simulink model "mech_four_bar_stat"  (Simulink 7.1)
settings: Solver=ode45  StartTime=0.0  StopTime=10.0  RelTol=1e-3  AbsTol=1e-3
libraries: mblibv1 x12
settings Model: Creator=paulk  LastModifiedBy=batserve  ExtModeAutoUpdateStatusClock=off
settings DataIOCC: SignalLoggingName=sigsOut
settings OptimizationCC: BooleanDataType=off  InlineInvariantSignals=on
settings DebuggingCC: SaveWithParameterizedLinksMsg=none  CheckExecutionContextPreStartOutputMsg=on  CheckExecutionContextRuntimeOutputMsg=on  SignalResolutionControl=TryResolveAllWithWarning  SolverPrmCheckMsg=none  MultiTaskDSMMsg=warning  MultiTaskCondExecSysMsg=none  StrictBusMsg=None
settings HardwareCC: TargetBitPerLong=64  TargetEndianess=LittleEndian  TargetWordSize=64  TargetHWDeviceType=MATLAB Host  ProdEqTarget=off
settings RTWCC: SystemTargetFile=rsim.tlc  TemplateMakefile=rsim_default_tmf  Description=Rapid Simulation Target  ProcessScript=rsim_make_rtw_hook  IncludeERTFirstTime=on
settings RSimTargetCC: TargetFcnLib=ansi_tfl_tmw.mat  TargetFunctionLibrary=ANSI_C  IsPILTarget=off  EnableShiftOperators=on  PortableWordSizes=off
settings SimMechanicsCC: WarnOnRedundantConstraints=off  VisOnUpdateDiagram=on  VisDuringSimulation=on

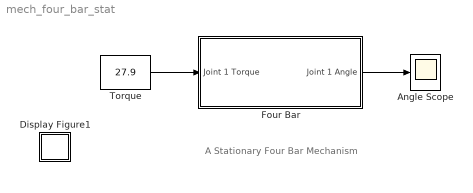
== system mech_four_bar_stat ==
  note: A Stationary Four Bar Mechanism
  Angle Scope : Scope
      settings: TimeRange=10  YMax=25
  Display Figure1 : Subsystem  Tag=Help  Description="Help callback for kinematic four bar model: mech_four_bar_kin.  Opens Help browser to Type 19 marker at documentation for this tutorial model."
      settings: OpenFcn=helpview([docroot '/toolbox/physmod/mech/mech.map'], 'mech_four_bar_stat_help');
      mask Type: Help callback
      mask Display: image(imread('info.bmp'))
  Four Bar : Subsystem
  Torque : Constant  Value=27.9  OutDataType=sfix(16)  OutScaling=2^0
  wires:
  Torque/1 -> Four Bar/1(Joint 1 Torque)
  Four Bar/1(Joint 1 Angle) -> Angle Scope/1

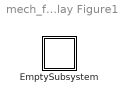
== system mech_four_bar_stat/Display Figure1 ==
  EmptySubsystem : Subsystem

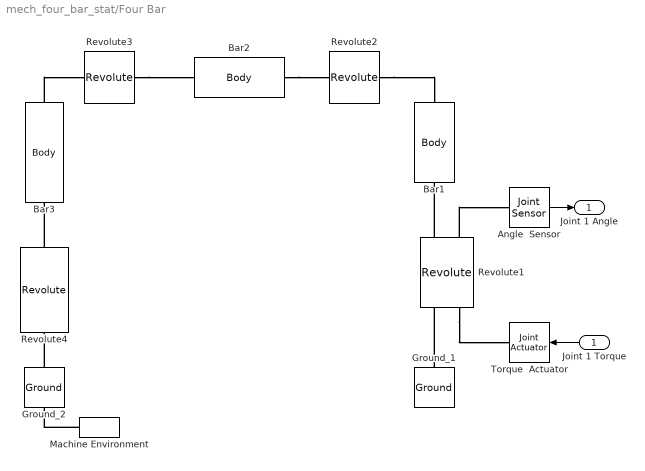
== system mech_four_bar_stat/Four Bar ==
  Joint 1 Torque : Inport  Orientation=left  OutDataType=sfix(16)  OutScaling=2^0
  Angle  Sensor : mblibv1/Sensors &  Actuators/Joint Sensor  DialogController=MECH.DynMechDlgSource  SystemSampleTime=-1  PhysicalDomain=Mechanical  PortType=blob  Muxed=on  Pose=off  Angle=on  AngleUnits=deg  ArcVelocity=off  ArcVelocityUnits=deg/s  ArcAcceleration=off  ArcAccelerationUnits=deg/s^2  CoordPosition=on  CoordPositionUnits=m  Velocity=off  VelocityUnits=m/s  Acceleration=off  AccelerationUnits=m/s^2  Quaternion=on  QuaternionDT=off  QuaternionDDT=off  QuaternionUnits=off  OutputVector=[ 1 ]  ActiveIO=on  Width=1  DialogClass=MechanicalSensorBlock  Primitive=R1  Force=off  ForceUnits=N  Torque=off  TorqueUnits=N-m  ReferenceFrame=Absolute (INERTIAL)  ReactionSensedSide=Base  ReactionReferenceFrame=Absolute (World)  ReactionForce=off  ReactionForceUnits=N  ReactionMoment=off  ReactionMomentUnits=N-m
  Bar1 : mblibv1/Bodies/Body  Orientation=up  DialogController=MECH.DynMechDlgSource  PhysicalDomain=mechanical  SubClassName=Unknown  LeftPortType=workingframe  RightPortType=workingframe  LConnTagsString=CS1  RConnTagsString=CS2  DialogClass=MechanicalBodyBlock  Mass=5.357  MassUnits=kg  InertiaUnits=kg*m^2  Inertia=[1.07e-3 0 0; 0 0.143 0;0 0 0.143]  Shape=Cylinder  ShapeDims=[1 1]  ShapeUnits=m  ShapeUse=false  Density=1  DensityUnits=kg/m^3  DensityUse=false  GraphicsMode=1  BodyColor=[0.5 0.5 0.5]  GraphicsObj=[]  AttachedToCS=1  CG=Left$CG$[0.03 0.282 0]$WORLD$CS1$m$[0 0 83.1]$Euler X-Y-Z$deg$WORLD$false  WorkingFrames=Left$CS1$[0 0 0]$WORLD$ADJOINING$m$[0 0 0]$Euler X-Y-Z$deg$WORLD$true#Right$CS2$[0.063 0.597 0]$WORLD$CS1$m$[0 0 0]$Euler X-Y-Z$deg$WORLD$true  CGPos=[0.03 0.282 0]  CGRot=[0 0 83.1]  CS0Pos=[]  CS0Rot=[]  CS1Pos=[0 0 0]  CS1Rot=[0 0 0]  CS2Pos=[0.063 0.597 0]  CS2Rot=[0 0 0]  CS3Pos=[]  CS3Rot=[]  CS4Pos=[]  CS4Rot=[]  CS5Pos=[]  CS5Rot=[]  CS6Pos=[]  CS6Rot=[]  CS7Pos=[]  CS7Rot=[]  CS8Pos=[]  CS8Rot=[]  CS9Pos=[]  CS9Rot=[]  CS10Pos=[]  CS10Rot=[]  CS11Pos=[]  CS11Rot=[]  CS12Pos=[]  CS12Rot=[]  CS13Pos=[]  CS13Rot=[]  CS14Pos=[]  CS14Rot=[]  CS15Pos=[]  CS15Rot=[]  CS16Pos=[]  CS16Rot=[]  CS17Pos=[]  CS17Rot=[]  CS18Pos=[]  CS18Rot=[]  CS19Pos=[]  CS19Rot=[]  CS20Pos=[]  CS20Rot=[]
  Bar2 : mblibv1/Bodies/Body  Orientation=left  DialogController=MECH.DynMechDlgSource  PhysicalDomain=mechanical  SubClassName=Unknown  LeftPortType=workingframe  RightPortType=workingframe  LConnTagsString=CS1  RConnTagsString=CS2  DialogClass=MechanicalBodyBlock  Mass=9.028  MassUnits=kg  InertiaUnits=kg*m^2  Inertia=[1.8e-3 0 0; 0 0.678 0;0 0 0.678]  Shape=Cylinder  ShapeDims=[1 1]  ShapeUnits=m  ShapeUse=false  Density=1  DensityUnits=kg/m^3  DensityUse=false  GraphicsMode=1  BodyColor=[0.5 0.5 0.5]  GraphicsObj=[]  AttachedToCS=1  CG=Left$CG$[-0.427 -0.242 0]$WORLD$CS1$m$[0 0 29.5]$Euler X-Y-Z$deg$WORLD$false  WorkingFrames=Left$CS1$[0 0 0]$WORLD$ADJOINING$m$[0 0 0]$Euler X-Y-Z$deg$WORLD$true#Right$CS2$[-0.87 -0.493 0]$WORLD$CS1$m$[0 0 0]$Euler X-Y-Z$deg$WORLD$true  CGPos=[-0.427 -0.242 0]  CGRot=[0 0 29.5]  CS0Pos=[]  CS0Rot=[]  CS1Pos=[0 0 0]  CS1Rot=[0 0 0]  CS2Pos=[-0.87 -0.493 0]  CS2Rot=[0 0 0]  CS3Pos=[]  CS3Rot=[]  CS4Pos=[]  CS4Rot=[]  CS5Pos=[]  CS5Rot=[]  CS6Pos=[]  CS6Rot=[]  CS7Pos=[]  CS7Rot=[]  CS8Pos=[]  CS8Rot=[]  CS9Pos=[]  CS9Rot=[]  CS10Pos=[]  CS10Rot=[]  CS11Pos=[]  CS11Rot=[]  CS12Pos=[]  CS12Rot=[]  CS13Pos=[]  CS13Rot=[]  CS14Pos=[]  CS14Rot=[]  CS15Pos=[]  CS15Rot=[]  CS16Pos=[]  CS16Rot=[]  CS17Pos=[]  CS17Rot=[]  CS18Pos=[]  CS18Rot=[]  CS19Pos=[]  CS19Rot=[]  CS20Pos=[]  CS20Rot=[]
  Bar3 : mblibv1/Bodies/Body  Orientation=down  DialogController=MECH.DynMechDlgSource  PhysicalDomain=mechanical  SubClassName=Unknown  LeftPortType=workingframe  RightPortType=workingframe  LConnTagsString=CS1  RConnTagsString=CS2  DialogClass=MechanicalBodyBlock  Mass=0.991  MassUnits=kg  InertiaUnits=kg*m^2  Inertia=[2.06e-4 0 0; 0 1.1e-3 0;0 0 1.1e-3]  Shape=Cylinder  ShapeDims=[1 1]  ShapeUnits=m  ShapeUse=false  Density=1  DensityUnits=kg/m^3  DensityUse=false  GraphicsMode=1  BodyColor=[0.5 0.5 0.5]  GraphicsObj=[]  AttachedToCS=1  CG=Left$CG$[-0.027 -0.048 0]$WORLD$CS1$m$[0 0 60]$Euler X-Y-Z$deg$WORLD$false  WorkingFrames=Left$CS1$[0 0 0]$WORLD$ADJOINING$m$[0 0 0]$Euler X-Y-Z$deg$WORLD$true#Right$CS2$[0 0 0]$WORLD$ADJOINING$m$[0 0 0]$Euler X-Y-Z$deg$WORLD$true  CGPos=[-0.027 -0.048 0]  CGRot=[0 0 60]  CS0Pos=[]  CS0Rot=[]  CS1Pos=[0 0 0]  CS1Rot=[0 0 0]  CS2Pos=[0 0 0]  CS2Rot=[0 0 0]  CS3Pos=[]  CS3Rot=[]  CS4Pos=[]  CS4Rot=[]  CS5Pos=[]  CS5Rot=[]  CS6Pos=[]  CS6Rot=[]  CS7Pos=[]  CS7Rot=[]  CS8Pos=[]  CS8Rot=[]  CS9Pos=[]  CS9Rot=[]  CS10Pos=[]  CS10Rot=[]  CS11Pos=[]  CS11Rot=[]  CS12Pos=[]  CS12Rot=[]  CS13Pos=[]  CS13Rot=[]  CS14Pos=[]  CS14Rot=[]  CS15Pos=[]  CS15Rot=[]  CS16Pos=[]  CS16Rot=[]  CS17Pos=[]  CS17Rot=[]  CS18Pos=[]  CS18Rot=[]  CS19Pos=[]  CS19Rot=[]  CS20Pos=[]  CS20Rot=[]
  Ground_1 : mblibv1/Bodies/Ground  Orientation=up  DialogController=MECH.DynMechDlgSource  SystemSampleTime=-1  LeftPortType=env  RightPortType=workingframe  PhysicalDomain=Mechanical  DialogClass=GroundBlock  CoordPosition=[0.434 0.04 0]  CoordPositionUnits=m  StateVectorMgrId=-1  MachineId=[0 0]  ShowEnvPort=off
  Ground_2 : mblibv1/Bodies/Ground  Orientation=up  DialogController=MECH.DynMechDlgSource  SystemSampleTime=-1  LeftPortType=env  RightPortType=workingframe  PhysicalDomain=Mechanical  DialogClass=GroundBlock  CoordPosition=[-0.433 0.04 0]  CoordPositionUnits=m  StateVectorMgrId=-1  MachineId=[0 0]  ShowEnvPort=on
  Machine Environment : mblibv1/Bodies/Machine Environment  Tag=Factory ground  Orientation=left  DialogController=MECH.DialogSource  SystemSampleTime=-1  PortType=env  PhysicalDomain=Mechanical  DialogTemplateClass=MECH.MachineEnvironment  SyncWhenCopied=off  Gravity=[0 -9.81 0]  GravityUnits=m/s^2  GravityAsSignal=off  Dimensionality=3D Only  AnalysisType=Forward dynamics  LinearAssemblyTolerance=1e-3  LinearAssemblyToleranceUnits=m  AngularAssemblyTolerance=1e-3  AngularAssemblyToleranceUnits=rad  ConstraintSolverType=Tolerancing  ConstraintRelTolerance=1e-4  ConstraintAbsTolerance=1e-4  UseRobustSingularityHandling=off  RedundancyAnalysisToleranceType=Automatically select tolerance  RedundancyAnalysisTolerance=1e-14  StatePerturbationType=Adaptive  PerturbationSize=0  VisualizeMachine=on
  Revolute1 : mblibv1/Joints/Revolute  Orientation=up  DialogController=MECH.DynMechDlgSource  PhysicalDomain=mechanical  SubClassName=Unknown  LeftPortType=blob  RightPortType=blob  LConnTagsString=__newl0|SA1  RConnTagsString=__newr0|SA1  NumSAPorts=2  CutJoint=off  MarkAsCut=off  Primitives=revolute  PrimitiveProps=R1$WORLD$[0 0 1]$revolute  DialogClass=JointBlock  R1Axis=[0 0 1]
  Revolute2 : mblibv1/Joints/Revolute  Orientation=left  DialogController=MECH.DynMechDlgSource  PhysicalDomain=mechanical  SubClassName=Unknown  LeftPortType=blob  RightPortType=blob  LConnTagsString=__newl0  RConnTagsString=__newr0  NumSAPorts=0  CutJoint=off  MarkAsCut=off  Primitives=revolute  PrimitiveProps=R1$WORLD$[0 0 1]$revolute  DialogClass=JointBlock  R1Axis=[0 0 1]
  Revolute3 : mblibv1/Joints/Revolute  Orientation=left  DialogController=MECH.DynMechDlgSource  PhysicalDomain=mechanical  SubClassName=Unknown  LeftPortType=blob  RightPortType=blob  LConnTagsString=__newl0  RConnTagsString=__newr0  NumSAPorts=0  CutJoint=off  MarkAsCut=off  Primitives=revolute  PrimitiveProps=R1$WORLD$[0 0 1]$revolute  DialogClass=JointBlock  R1Axis=[0 0 1]
  Revolute4 : mblibv1/Joints/Revolute  Orientation=down  DialogController=MECH.DynMechDlgSource  PhysicalDomain=mechanical  SubClassName=Unknown  LeftPortType=blob  RightPortType=blob  LConnTagsString=__newl0  RConnTagsString=__newr0  NumSAPorts=0  CutJoint=off  MarkAsCut=off  Primitives=revolute  PrimitiveProps=R1$WORLD$[0 0 1]$revolute  DialogClass=JointBlock  R1Axis=[0 0 1]
  Torque  Actuator : mblibv1/Sensors &  Actuators/Joint Actuator  Orientation=left  DialogController=MECH.DynMechDlgSource  SystemSampleTime=-1  PhysicalDomain=Mechanical  PortType=blob  ActuationStyle=Force  AngleUnits=deg  ArcVelocityUnits=deg/s  ArcAccelerationUnits=deg/s^2  CoordPositionUnits=m  VelocityUnits=m/s  AccelerationUnits=m/s^2  ForceUnits=N  TorqueUnits=N-m  ActiveIO=on  Width=1  DialogClass=MechanicalActuatorBlock  Primitive=R1  ReferenceFrame=Absolute (INERTIAL)
  Joint 1 Angle : Outport  OutDataType=sfix(16)  OutScaling=2^0
  wires:
  Joint 1 Torque/1 -> Torque  Actuator/1
  Angle  Sensor/1 -> Joint 1 Angle/1
  connections:
  Revolute3/LConn1 -- Bar2/RConn1
  Bar2/LConn1 -- Revolute2/RConn1
  Revolute2/LConn1 -- Bar1/RConn1
  Revolute1/RConn1 -- Bar1/LConn1
  Ground_1/RConn1 -- Revolute1/LConn1
  Bar3/LConn1 -- Revolute3/RConn1
  Revolute4/LConn1 -- Bar3/RConn1
  Ground_2/RConn1 -- Revolute4/RConn1
  Revolute1/LConn2 -- Torque  Actuator/RConn1
  Revolute1/RConn2 -- Angle  Sensor/LConn1
  Machine Environment/RConn1 -- Ground_2/LConn1

== system mech_four_bar_stat/Display Figure1/EmptySubsystem ==
